simulink model "AeroBenchSim"  (R2017b)
settings: Solver=VariableStepAuto  StartTime=0.0  StopTime=10.0  RelTol=1e-3
InitFcn:
  | % Add simulink directory to MATLAB Path
  | filepath=get_param(gcs, 'filename');
  | sim_dir = fileparts(filepath);
  | addpath(genpath(sim_dir))
  | 
  | % Configure workspace for sim
  | SimConfig;
settings Model: Creator=HeidlaPT  LastModifiedBy=HeidlaPT

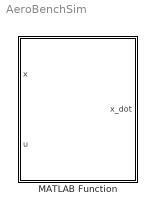
== system AeroBenchSim ==
  MATLAB Function : MATLAB Function  Tag=F-16  Description=Given aircraft state and raw control inputs, uses subf16_morelli to generate aircraft state derivatives  TreatAsAtomicUnit=on

== matlab function AeroBenchSim/MATLAB Function ==
  data: x input; u input; x_dot output
function x_dot = F16_plant(x,u)
[x_dot, Nz, Ny] = subf16_morelli(x,u);
